simulink model "observer_model"  (R2024b)
settings: Solver=VariableStepAuto  StartTime=0.0  StopTime=10.0  RelTol=1e-3
values from neighbouring files (symbols this model uses):
  A = [0,1; 0,-10]    [conti_ss_script.m]    (also in discrete_script.m = [0,1; -3, -60]; error_space_script.m = [0,1; 0,-20]; observer_script.m = [0,1; 0,-20]; pid_script.m)
  AobsFull = A-Lfull*C    [observer_script.m]
  AobsRed = A(2,2)-Lred*A(1,2)    [observer_script.m]
  B = [0; 120]    [conti_ss_script.m]    (also in discrete_script.m = [0; 1]; error_space_script.m = [0; 60]; observer_script.m = [0; 60]; pid_script.m)
  BobsFull = [B, Lfull]    [observer_script.m]
  BobsRed = [B(2)-Lred*B(1), AobsRed*Lred+A(2,1)-Lred*A(1,1)]    [observer_script.m]
  C = [1, 0]    [conti_ss_script.m]    (also in discrete_script.m = [90, 0]; error_space_script.m = [1,0]; observer_script.m = [1,0]; pid_script.m)
  CobsFull = eye(2)    [observer_script.m]
  CobsRed = [0;1]    [observer_script.m]
  D = 0    [conti_ss_script.m]    (also in discrete_script.m; error_space_script.m; observer_script.m; pid_script.m)
  DobsFull = zeros(2)    [observer_script.m]
  DobsRed = [0,1; 0,Lred]    [observer_script.m]
  K = Ke(2:end)    [conti_ss_script.m]    (also in discrete_script.m = Kdd; error_space_script.m = Kz(4:5); observer_script.m)
  Ki = Ke(1)    [conti_ss_script.m]    (also in observer_script.m; pid_script.m = -w_gc * dK*sin(dphi))
  Nu = ff(3)    [conti_ss_script.m]    (also in discrete_script.m = Nudd; observer_script.m)
  Nx = ff(1:2)    [conti_ss_script.m]    (also in discrete_script.m = Nxdd; observer_script.m)
settings Model: Creator=pries  LastModifiedBy=pries

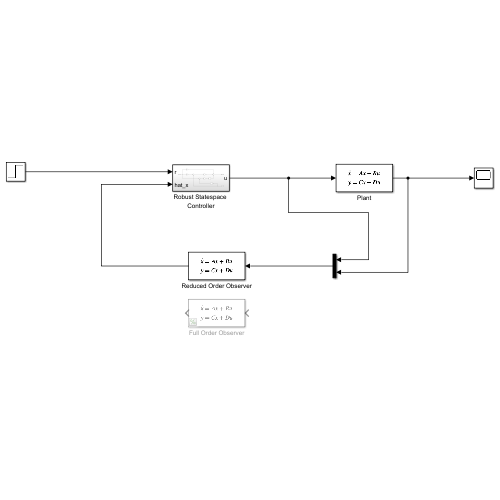
[thumbnail: Simulink's stored preview of the top-level diagram]
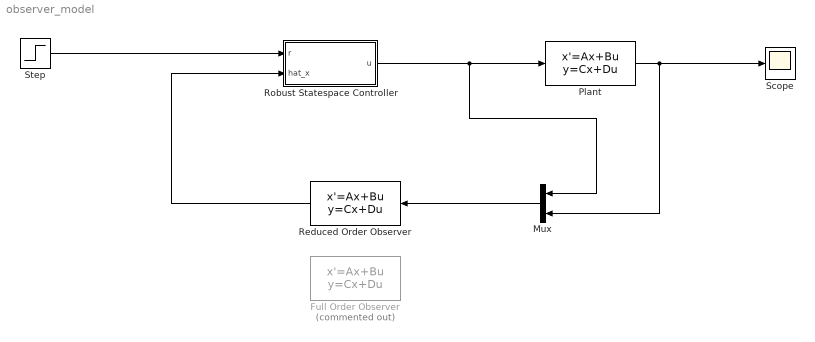
== system observer_model ==
  Full Order Observer : StateSpace  Commented=on  A=AobsFull  B=BobsFull  C=CobsFull  D=DobsFull  InitialCondition=0
  Mux : Mux  Inputs=2
  Plant : StateSpace  A=A  B=B  C=C  D=D  InitialCondition=0
  Reduced Order Observer : StateSpace  A=AobsRed  B=BobsRed  C=CobsRed  D=DobsRed  InitialCondition=0
  Robust Statespace Controller : Subsystem
  Scope : Scope
  Step : Step  SampleTime=0
  wires:
  Robust Statespace Controller/1(u) -> Plant/1, Mux/1
  Mux/1 -> Reduced Order Observer/1
  Plant/1 -> Scope/1, Mux/2
  Reduced Order Observer/1 -> Robust Statespace Controller/2(hat_x)
  Step/1 -> Robust Statespace Controller/1(r)

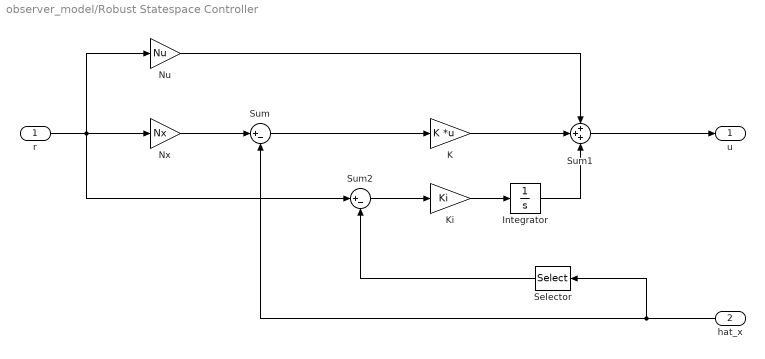
== system observer_model/Robust Statespace Controller ==
  r : Inport
  hat_x : Inport  Port=2
  Integrator : Integrator
  K : Gain  Gain=K  Multiplication=Matrix(K*u)
  Ki : Gain  Gain=Ki
  Nu : Gain  Gain=Nu
  Nx : Gain  Gain=Nx
  Selector : Selector  InputPortWidth=2  IndexOptions=Index vector (dialog)  Indices=1  OutputSizes=1
  Sum : Sum  Inputs=|+-
  Sum1 : Sum  Inputs=+++
  Sum2 : Sum  Inputs=|+-
  u : Outport
  wires:
  r/1 -> Sum2/1, Nu/1, Nx/1
  Nx/1 -> Sum/1
  Sum/1 -> K/1
  Nu/1 -> Sum1/1
  K/1 -> Sum1/2
  Sum1/1 -> u/1
  hat_x/1 -> Selector/1, Sum/2
  Ki/1 -> Integrator/1
  Integrator/1 -> Sum1/3
  Sum2/1 -> Ki/1
  Selector/1 -> Sum2/2
